simulink model "robosimppi"  (R2021a)
settings: Solver=ode45  StartTime=0.0  StopTime=50  MaxStep=0.1  RelTol=1e-4  EnableMultiTasking=on
values from neighbouring files (symbols this model uses):
  kd = [400*bar_m11 0; 0 400*bar_m22]    [mppi.m]    (also in pd.m = [4000.2 0; 0 52200]; slotine.m = 10*[Il1+Ml1*l1^2+(Kr1^2)*Im1+Il2+Ml2*(a(1)^2+l2^2)+Im2+Mm2*a; tcpd.m = [20 0; 0 20])
  ki = [4e4*bar_m11 0;0 4e4*bar_m22]    [mppi.m]
  kp = [19.75 0;0 19.75]    [mppi.m]    (also in pd.m = [20001 0;0 261000]; tcpd.m = [100 0;0 100])
  q0 = [pi/4  -pi/2 0 0]    [mpd.m]    (also in mppi.m = [pi/4 -pi/2 0 0]; mslotine.m; mtcpd.m)
  traj = 1    [mpd.m]    (also in mppi.m; mslotine.m; mtcpd.m; pd.m)
settings Model: ExtModeAutoUpdateStatusClock=off  Creator=fernando  LastModifiedBy=Guga
settings SolverCC: AlgebraicLoopSolver=TrustRegion
settings DataIOCC: LimitDataPoints=on  SaveFormat=Array  SignalLoggingSaveFormat=ModelDataLogs
settings OptimizationCC: ExpressionDepthLimit=2147483647  InitFltsAndDblsToZero=on  LifeSpan=inf
settings DebuggingCC: SaveWithParameterizedLinksMsg=none  UnderspecifiedInitializationDetection=Classic  MergeDetectMultiDrivingBlocksExec=none  SignalResolutionControl=TryResolveAllWithWarning  SolverPrmCheckMsg=warning  MultiTaskDSMMsg=warning  MultiTaskCondExecSysMsg=none  FcnCallInpInsideContextMsg=warning  StateNameClashWarn=warning  SFUnexpectedBacktrackingDiag=warning  SFNoUnconditionalDefaultTransitionDiag=warning  SFExecutionAtInitializationDiag=none  SFMachineParentedDataDiag=warning  ArithmeticOperatorsInVariantConditions=warning
settings HardwareCC: ProdBitPerPointer=32  ProdBitPerSizeT=32  ProdBitPerPtrDiffT=32  ProdLargestAtomicFloat=None  ProdIntDivRoundTo=Undefined  ProdEndianess=Unspecified  ProdWordSize=32  ProdHWDeviceType=32-bit Generic
settings ModelReferenceCC: PropagateSignalLabelsOutOfModel=off
settings SFSimCC: SimUseLocalCustomCode=off  SimParseCustomCode=off  CustomCodeUndefinedFunction=UseInterfaceOnly
settings RTWCC: RTWUseLocalCustomCode=off
settings CodeAppCC: StateflowObjectComments=on
settings GRTTargetCC: TargetFcnLib=ansi_tfl_tmw.mat  TargetLangStandard=C89/C90 (ANSI)  CombineOutputUpdateFcns=off  GRTInterface=on
settings ConfigComp: CovMetricSettings=dw  CovSaveCumulativeToWorkspaceVar=on  CovSaveSingleToWorkspaceVar=on  CovExternalEMLEnable=off

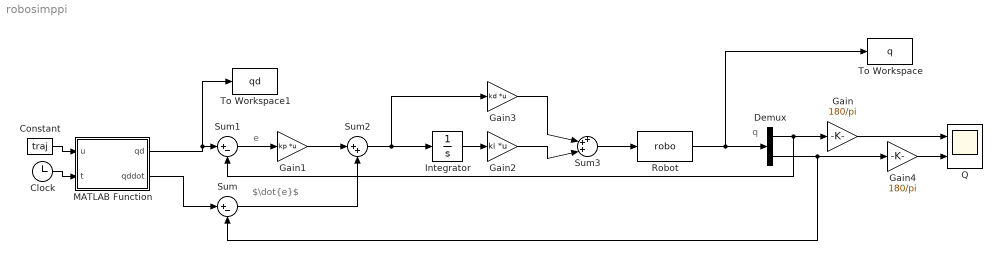
== system robosimppi ==
  note: e
  note: q
  note: $\dot{e}$
  Clock : Clock
  Constant : Constant  Value=traj
  Demux : Demux  Outputs=2
  Gain : Gain  Gain=180/pi
  Gain1 : Gain  Gain=kp  Multiplication=Matrix(K*u)
  Gain2 : Gain  Gain=ki  Multiplication=Matrix(K*u)
  Gain3 : Gain  Gain=kd  Multiplication=Matrix(K*u)
  Gain4 : Gain  Gain=180/pi
  Integrator : Integrator  InitialCondition=[pi/4; -pi/2]
  MATLAB Function : MATLAB Function  TreatAsAtomicUnit=on
  Q : Scope  NumInputPorts=2
  Robot : S-Function  FunctionName=robo  Parameters=q0  SFunctionDeploymentMode=off  EnableBusSupport=off  mask(Robot){xi=q0}
      mask prompts: xi "Condicao Inicial"
  Sum : Sum  Inputs=|+-
  Sum1 : Sum  Inputs=|+-
  Sum2 : Sum  Inputs=|++
  Sum3 : Sum  Inputs=+++|
  To Workspace : ToWorkspace  VariableName=q  SaveFormat=Timeseries  SampleTime=-1
  To Workspace1 : ToWorkspace  VariableName=qd  SaveFormat=Timeseries  SampleTime=-1
  wires:
  Demux/2 -> Gain4/1, Sum/2
  Demux/1 -> Sum1/2, Gain/1
  Robot/1 -> Demux/1, To Workspace/1
  Constant/1 -> MATLAB Function/1(u)
  Clock/1 -> MATLAB Function/2(t)
  MATLAB Function/1(qd) -> To Workspace1/1, Sum1/1
  MATLAB Function/2(qddot) -> Sum/1
  Sum1/1 -> Gain1/1
  Sum/1 -> Sum2/2
  Gain1/1 -> Sum2/1
  Sum2/1 -> Gain3/1, Integrator/1
  Integrator/1 -> Gain2/1
  Gain3/1 -> Sum3/2
  Gain2/1 -> Sum3/3
  Sum3/1 -> Robot/1
  Gain/1 -> Q/1
  Gain4/1 -> Q/2

== matlab function robosimppi/MATLAB Function ==
  data: u input; qd output; qddot output; t input
function [qd,qddot] = fcn(u,t)
switch u
    case 1 % rapida
        qd1= -0.75*cos(pi*t)-0.75;
        qd2= -0.75*cos(1.2*pi*t)+3.75;
        dt1 = 0.75*sin(pi*t)*pi;
        dt2 = 0.75*sin(1.2*pi*t)*1.2*pi;
    case 2 % lenta
        qd1= -0.75*cos((pi/2)*t)-0.75;
        qd2= -0.75*cos((1.2/2)*pi*t)+3.75;
        dt1 = 0.75*sin((pi/2)*t)*pi/2;
        dt2 = 0.75*sin((1.2/2)*pi*t)*(1.2/2)*pi;
    otherwise 
        qd1 = 1 + 0*t;
        qd2 = qd1;
        dt1 = 0 + 0*t;
        dt2 = dt1;
    
end

qd = [qd1; qd2];
qddot = [dt1;dt2];
end
